simulink model "ADPSEStaF3DOldEMK"  (R2018b)
settings: Solver=ode1  StartTime=0.0  StopTime=100  FixedStep=1/1000  RelTol=1e-3  AbsTol=1e-3  EnableMultiTasking=on
PostLoadFcn:
  | f_Simulink_figureplace
InitFcn:
  | ADPSEStaF3DOldEMK_PreSim
values from neighbouring files (symbols this model uses):
  beta = 0.0001    [ADPSEStaF3DOldEMK_PreSim.m]
  D = 0    [ADPSEStaF3DOldEMK_PreSim.m]
  dbar = 0.0    (= 0)    [ADPSEStaF3DOldEMK_PreSim.m]
  etaa1 = 17    [ADPSEStaF3DOldEMK_PreSim.m]
  etaa2 = 0.001    [ADPSEStaF3DOldEMK_PreSim.m]
  etac1 = 0.001    [ADPSEStaF3DOldEMK_PreSim.m]
  etac2 = 20    [ADPSEStaF3DOldEMK_PreSim.m]
  Gamma0 = 100*eye(L)    [ADPSEStaF3DOldEMK_PreSim.m]
  MovePoints = 0    [ADPSEStaF3DOldEMK_PreSim.m]
  NormBas = 0    [ADPSEStaF3DOldEMK_PreSim.m]
  NormDyn = 0    [ADPSEStaF3DOldEMK_PreSim.m]
  Q = 10*eye(n)    [ADPSEStaF3DOldEMK_PreSim.m]
  R = eye(m)    [ADPSEStaF3DOldEMK_PreSim.m]
  s = 1    [ADPSEStaF3DOldEMK_PreSim.m]
  v = 0.5    [ADPSEStaF3DOldEMK_PreSim.m]
  v2 = 2    [ADPSEStaF3DOldEMK_PreSim.m]
  WaH0 = 0.85*WcH0    [ADPSEStaF3DOldEMK_PreSim.m]
  WcH0 = 1*ones(L,1)    [ADPSEStaF3DOldEMK_PreSim.m]
  x0 = [-0.5; 0.5; -0.250]    [ADPSEStaF3DOldEMK_PreSim.m]
settings Model: Creator=rkamalapurkar  LastModifiedBy=rushik
settings SolverCC: AutoScaleAbsTol=off
settings DataIOCC: SaveFormat=StructureWithTime  SaveOutput=off  DSMLogging=off  SaveTime=off  SignalLoggingName=ADPCLStaF
settings OptimizationCC: ExpressionDepthLimit=2147483647  LifeSpan=inf
settings DebuggingCC: UnderspecifiedInitializationDetection=Classic  MergeDetectMultiDrivingBlocksExec=none  SolverPrmCheckMsg=warning  FcnCallInpInsideContextMsg=warning  StateNameClashWarn=warning  SFUnexpectedBacktrackingDiag=warning  SFNoUnconditionalDefaultTransitionDiag=warning  SFExecutionAtInitializationDiag=none
settings HardwareCC: ProdBitPerPointer=32  ProdBitPerSizeT=32  ProdBitPerPtrDiffT=32  ProdLargestAtomicFloat=None  ProdIntDivRoundTo=Undefined  ProdEndianess=Unspecified  ProdWordSize=32  ProdHWDeviceType=32-bit Generic
settings ModelReferenceCC: PropagateSignalLabelsOutOfModel=off
settings SFSimCC: SimUseLocalCustomCode=off
settings RTWCC: RTWUseLocalCustomCode=off
settings CodeAppCC: StateflowObjectComments=on
settings GRTTargetCC: TargetLangStandard=C89/C90 (ANSI)  GeneratePreprocessorConditionals=Disable all  CombineOutputUpdateFcns=off  GRTInterface=on
settings ConfigComp: CovMetricSettings=dw  CovHtmlReporting=on  CovSaveCumulativeToWorkspaceVar=on  CovSaveSingleToWorkspaceVar=on  CovExternalEMLEnable=off  CovSFcnEnable=off

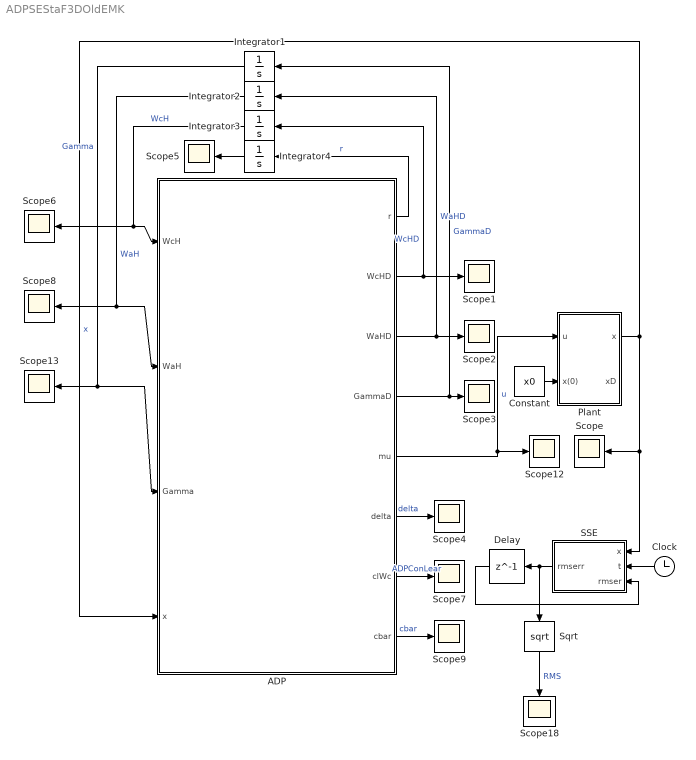
== system ADPSEStaF3DOldEMK ==
  ADP : MATLAB Function  TreatAsAtomicUnit=on
  Clock : Clock
  Constant : Constant  Value=x0
  Delay : Delay  DelayLength=1  InitialCondition=0
  Integrator1 : Integrator  InitialCondition=Gamma0
  Integrator2 : Integrator  InitialCondition=WaH0
  Integrator3 : Integrator  InitialCondition=WcH0
  Integrator4 : Integrator
  Plant : Subsystem
  SSE : MATLAB Function  TreatAsAtomicUnit=on
  Scope{,1..9,12..13,18} (13 alike) : Scope
  Sqrt : Sqrt  SaturateOnIntegerOverflow=on
  wires:
  ADP/4(GammaD) -> Integrator1/1, Scope3/1  "GammaD"
  ADP/2(WcHD) -> Scope1/1, Integrator3/1  "WcHD"
  Integrator3/1 -> ADP/1(WcH), Scope6/1  "WcH"
  ADP/3(WaHD) -> Scope2/1, Integrator2/1  "WaHD"
  Integrator2/1 -> ADP/2(WaH), Scope8/1  "WaH"
  ADP/6(delta) -> Scope4/1  "delta"
  Integrator1/1 -> ADP/3(Gamma), Scope13/1  "Gamma"
  ADP/7(clWc) -> Scope7/1  "ADPConLear"
  Plant/1(x) -> ADP/4(x), SSE/1(x), Scope/1  "x"
  Constant/1 -> Plant/2(x(0))
  ADP/8(cbar) -> Scope9/1  "cbar"
  Clock/1 -> SSE/2(t)
  SSE/1(rmserr) -> Sqrt/1, Delay/1
  Delay/1 -> SSE/3(rmser)
  Sqrt/1 -> Scope18/1  "RMS"
  ADP/5(mu) -> Scope12/1, Plant/1(u)  "u"
  ADP/1(r) -> Integrator4/1  "r"
  Integrator4/1 -> Scope5/1

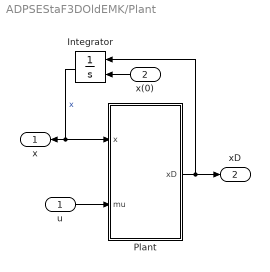
== system ADPSEStaF3DOldEMK/Plant ==
  u : Inport
  x(0) : Inport  Port=2
  Integrator : Integrator  InitialConditionSource=external  InitialCondition=[1;1;0.0;0.0]
  Plant : MATLAB Function  TreatAsAtomicUnit=on
  x : Outport
  xD : Outport  Port=2
  wires:
  Plant/1(xD) -> Integrator/1, xD/1
  Integrator/1 -> Plant/1(x), x/1  "x"
  u/1 -> Plant/2(mu)
  x(0)/1 -> Integrator/2

== matlab function ADPSEStaF3DOldEMK/Plant/Plant ==
  data: xD output; x input; mu input
function xD = dynamics(x,mu)
%#codegen
P = [1 1 1;
     0 1 1;
     0 0 1];
F = [x(2);x(3);sqrt(x'*P*x)];
G=[0 0; 1 0; 0 1];
xD = F+G*mu;

== matlab function ADPSEStaF3DOldEMK/ADP ==
  data: r output; WcH input; WaH input; Gamma input; x input; R parameter; Q parameter; etaa1 parameter; etaa2 parameter; v2 parameter; s parameter; dbar parameter; D parameter; etac1 parameter; etac2 parameter; v parameter; WcHD output; WaHD output; GammaD output; mu output; delta output; clWc output; beta parameter; MovePoints parameter; cbar output; NormBas parameter; NormDyn parameter; x0 parameter
function [r,WcHD,WaHD,GammaD,mu,delta,clWc,cbar]=...
    control(WcH,WaH,Gamma,x,R,Q,etaa1,etaa2,v2,s,dbar,D,...
    etac1,etac2,v,beta,MovePoints,NormBas,NormDyn,x0)
%#codegen

if NormDyn == 1
    a = norm(x0);
else
    a = 1;
end
n=3;
% thetaS=[-1 1 -0.5 -0.5]'; % True values of SysID Parameters
y = x/a;
G=[0 0; 1 0; 0 1]./a;
% Y = [a*y(1) a*y(2) 0 0;0 0 a*y(1) a*y(2)*(1-(cos(2*a*y(1))+2)^2)]./a;
P = [1 1 1;
     0 1 1;
     0 0 1];
F = [x(2);x(3);sqrt(x'*P*x)];
[sig,sig_p] = ADPSEStaF3DOldEMK_Basis(y);
mu=-0.5*(R\G')*sig_p'*WaH;

% theta = thetaS;%*(model==1) + thetaH*(model~=1);
%% Concurrent Learning
% nm=(y'*y+dbar)/(1+v2*(y'*y));
nm=1;
if MovePoints == 0
    temp=linspace(-4*s*nm,1*s*nm,4);
    [temp1, temp2, temp3] = ndgrid(temp,temp,temp);
    XC=[temp1(:) temp2(:) temp3(:)]'; % matrix with columns as selected points
    M = length(temp)^n; %Number of points
else
    M=1;
    XC=unifrnd(-3*s*nm,3*s*nm,n,M);
% XC1=sin(2*pi*t) + sin(exp(1)*t) + cos(5*t)^5;
% XC2=sin(5*pi*t) + sin(exp(8)*t) + cos(2*t)^5;
% XC3=sin(4*pi*t) + sin(exp(1.4)*t) + cos(1*t)^5;
% XC4=sin(5*pi*t) + sin(exp(1.3)*t) + cos(0.5*t)^5;
% XC5=sin(3*pi*t) + sin(exp(1.1)*t) + cos(10*t)^5;
% XC6=sin(2*pi*t) + sin(exp(1.8)*t) + cos(11*t)^5;
% XC=[XC1;XC2];
end
clWc=zeros(size(WcH));
clWa=zeros(size(WaH));
CLmatrix=zeros(size(WcH,1),size(WcH,1));
CLGamma=zeros(size(Gamma));
parfor i=1:M
    xi=XC(:,i);
    [~,sig_pi] = ADPSEStaF3DOldEMK_Basis(xi);   
    Gi=[0 0; 1 0; 0 1]./a;
%     Yi = [xi(1) xi(2) 0 0;0 0 xi(1) xi(2)*(1-(cos(2*xi(1))+2)^2)]./a;
    Fi = [xi(2);xi(3);sqrt(xi'*P*xi)];
    mui=-0.5*(R\Gi')*sig_pi'*WaH;
    omegai = sig_pi*(Fi+Gi*mui);
    rhoi=(1+v*(omegai'*omegai));
    ri = xi'*Q*xi*a^2 + mui'*R*mui;
    deltai = WcH'*omegai + ri;
    clWc=clWc+Gamma*omegai*deltai/rhoi;
    Gsigmai = sig_pi*Gi*(R\Gi')*sig_pi';
    clWa=clWa+Gsigmai'*WaH*omegai'*WcH/(4*rhoi);
    CLmatrix=CLmatrix+omegai*omegai'/(M*rhoi);
    CLGamma=CLGamma+Gamma*(omegai*omegai'/rhoi^2)*Gamma;
end
clWc=-etac2*clWc/M;
clWa=etac2*clWa/M;
CLGamma=CLGamma/M;
cbar=min(svd(CLmatrix));
%% ADP
omega = sig_p*(F+G*mu);
Gsigma = sig_p*G*(R\G')*sig_p';
r = y'*Q*y*a^2 + mu'*R*mu;
delta = WcH'*omega + r;
rho = (1+v*(omega'*omega));
WcHD = (-etac1*Gamma*omega*delta/rho+clWc);
GammaD = (beta*Gamma-Gamma*(omega*omega'/rho^2)*Gamma-CLGamma);
WaHD = etaa1*(WcH-WaH)...
    -(etaa2*WaH-etac1*Gsigma'*WaH*omega'*WcH/(4*rho))+clWa;

== matlab function ADPSEStaF3DOldEMK/SSE ==
  data: x input; t input; rmser input; rmserr output
function rmserr = fcn(x,t,rmser)
%#codegen

if t>90
    rmserr = rmser+(1/10000)*(norm(x))^2;
else
    rmserr = 0;
end
